simulink model "Loops5"  (Simulink 8.7)
settings: Solver=ode45  StartTime=0.0  StopTime=10.0  RelTol=1e-3
settings Model: Creator=scaife  LastModifiedBy=bourbouh  ExtModeAutoUpdateStatusClock=off
settings DataIOCC: SignalLoggingSaveFormat=ModelDataLogs  SignalLoggingName=sigsOut
settings OptimizationCC: InitFltsAndDblsToZero=on
settings DebuggingCC: SaveWithParameterizedLinksMsg=none  SignalResolutionControl=TryResolveAllWithWarning  MultiTaskDSMMsg=warning  MultiTaskCondExecSysMsg=none
settings HardwareCC: TargetUnknown=on
settings SFSimCC: SimParseCustomCode=off
settings GRTTargetCC: TargetFcnLib=ansi_tfl_tmw.mat  ModelReferenceCompliant=off  GeneratePreprocessorConditionals=Use local settings  CombineOutputUpdateFcns=off  MatFileLogging=off  GRTInterface=on

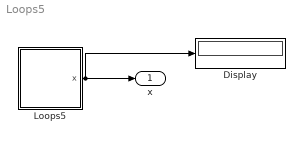
== system Loops5 ==
  Display : Display
  Loops5 : Stateflow chart  TreatAsAtomicUnit=on
  x : Outport
  wires:
  Loops5/1(x) -> x/1, Display/1

== stateflow chart Loops5 ==
  state A
  state B
  B -> A : {y=(y+1)%%2;}
  (default) -> A : {y=0;}
  A -> (junction 7) : {x=0;}
  (junction 8) -> (junction 7) [order 1] : [x<10]
      | {x++;}
  (junction 7) -> (junction 8) [order 2]
  (junction 7) -> (junction 9) [order 1] : [y==1]
  (junction 9) -> (junction 9) [order 1] : [x<5]
      | {x++;}
  (junction 8) -> B [order 2]
  (junction 9) -> B [order 2]
  data: x output int32; y local int32
